simulink model "GNSS_MPCcontrolledSpacecraft"  (R2025b)
settings: Solver=ode113  StartTime=0.0  StopTime=120  FixedStep=1*60*60  RelTol=1e-8  AbsTol=1e-8
values from neighbouring files (symbols this model uses):
  area = 15    [Script_Concurso_Spacecraft_batch.m]    (also in initialize_inoas_simulation.m = 0.03)
  initMass = m_sat    (= 10000)    [Script_Concurso_Spacecraft_batch.m]    (also in initialize_inoas_simulation.m = 3.99)
  lamda_init = 1    [initialize_inoas_simulation.m]
  m = cfg.m    [MPC_INOAS.m]    (also in Script_Concurso_Spacecraft_batch.m = 3; initialize_inoas_simulation.m = 3)
  ref = 1.3    [Script_Concurso_Spacecraft_batch.m]    (also in initialize_inoas_simulation.m = 1)
  s = [sigma_x,sigma_x,sigma_x,sigma_v,sigma_v,sigma_v]    [Script_Concurso_Spacecraft_batch.m]    (also in initialize_inoas_simulation.m = [sigma_x, sigma_x, sigma_x, sigma_v, sigma_v, sigma_v])
  S_inv = inv(S)    [Script_Concurso_Spacecraft_batch.m]    (also in initialize_inoas_simulation.m)
  S_T_inv = inv(S')    [Script_Concurso_Spacecraft_batch.m]    (also in initialize_inoas_simulation.m)
  Ts = 1    [Script_Concurso_Spacecraft_batch.m]    (also in initialize_inoas_simulation.m)
  var_alt = sigma_alt^2    (= 1)    [Script_Concurso_Spacecraft_batch.m]    (also in initialize_inoas_simulation.m = 4000000)
  var_IMU = 0.01    [Script_Concurso_Spacecraft_batch.m]
  var_pos = sigma_pos^2    (= 10000)    [Script_Concurso_Spacecraft_batch.m]    (also in initialize_inoas_simulation.m = 4000000)
undefined symbols (not defined in the file or in its folder): endDate, thrustingThreshold
libraries: simulink x6, vrlib x2, sharedTrackingLibrary x1, aerolibsatdyn x1, aerolibutil x1
settings Model: SimulationMode=accelerator  Creator=benit  LastModifiedBy=Enrique Valverde

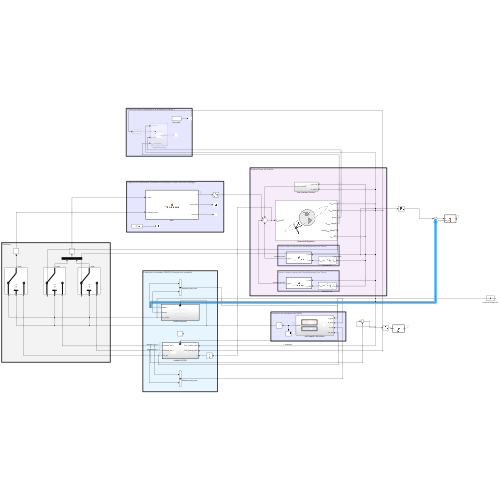
[thumbnail: Simulink's stored preview of the top-level diagram]
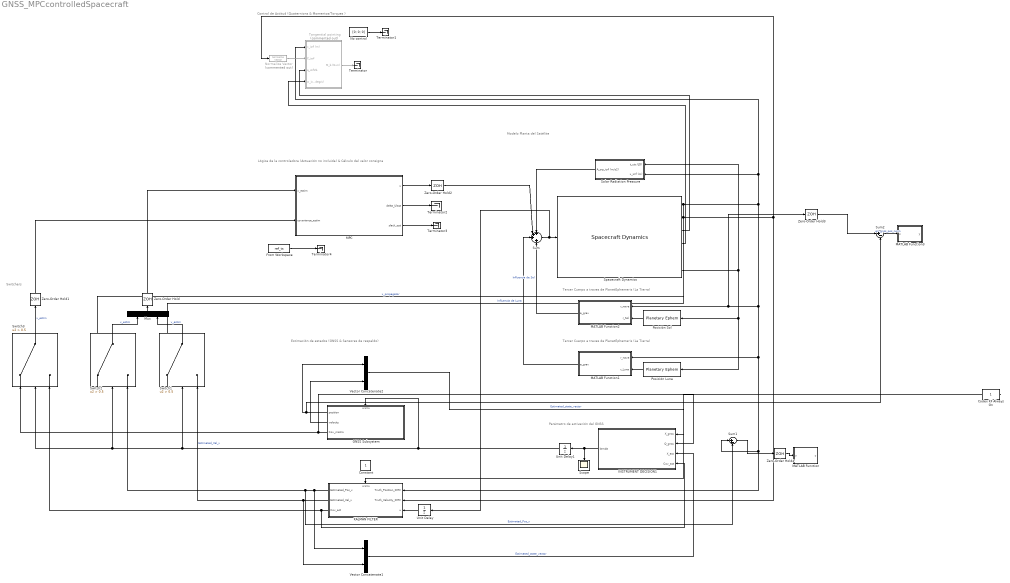
== system GNSS_MPCcontrolledSpacecraft ==
  note: Switchers
  note: Control de Actitud (Quaternions & Momentos/Torques )
  note: Lógica de la controladora (Actuación no incluida) & Cálculo del valor consigna
  note: Estimación de estados (GNSS & Sensores de respaldo)
  note: Parámetro de activación del GNSS
  note: Modelo Planta del Satélite
  note: Tercer Cuerpo a traves de PlanetEphemeris (La Tierra)
  note: Tercer Cuerpo a traves de PlanetEphemeris (La Tierra)
  Codex KF Always On : Constant  OutDataTypeStr=boolean
  Constant : Constant
  From Workspace : FromWorkspace  VariableName=ref_ts  SampleTime=1
  GNSS Subsystem : Subsystem  Description=|  TreatAsAtomicUnit=on
      | "GNSS ON"
      | 
      | Aquí va a ir las medidas del vector de estados utilizando GNSS. 
      | 
      | Se tendrá que añadir todo el sistema de ruido blanco del sensor, así como la regresión
      | por medio de mínimos cuadrados (WLSQ)
  INSTRUMENT DECISION1 : Subsystem
  KALMAN FILTER : Subsystem  Description=|  TreatAsAtomicUnit=on
      | "GNSS OFF"
      | 
      | Aquí va a ir las medidas del vector de estados utilizando Backup Sensor. 
      | 
      | Se tendrá que añadir todo el sistema de ruido blanco de los sensor de respaldo, 
      | así como el Filtro de Kalman y la estadística que permita mezclar las distintas medidas 
      | de distinta procedencia.
  MATLAB Function : MATLAB Function  TreatAsAtomicUnit=on
  MATLAB Function1 : MATLAB Function  TreatAsAtomicUnit=on
  MATLAB Function2 : MATLAB Function  TreatAsAtomicUnit=on
  MATLAB Function3 : MATLAB Function  TreatAsAtomicUnit=on
  MPC : MATLAB Function  TreatAsAtomicUnit=on
  Mux : Mux  Inputs=2
  No control : Constant  Value=[0; 0; 0]
  Normalize Vector : vrlib/Utilities/Normalize Vector  Commented=on  maxzero=0
  Posición Luna : PlanetaryEphem  units=m,m/s  center=Sun  startDate=startDate2  endDate=endDate*1.02  outputVelocity=off
  Posición Sol : PlanetaryEphem  units=m,m/s  target=Sun  startDate=startDate2  endDate=endDate*1.02  outputVelocity=off
  Scope : Scope
      settings: ActiveDisplayYMinimum=0.9  ActiveDisplayYMaximum=1.1
  Solar Radiation Pressure : Subsystem
  Spacecraft Dynamics : SpacecraftDynamics  forcesIn=off  momentsIn=off  accelIn=on  startDate=start_date  mass=m_sat  semiMajorAxis=a  eccentricity=ecc  inclination=inc  raan=RAAN  argPeriapsis=w  trueAnomaly=theta  outputAngAccel=on  shDegree=2  ephemerisStartDate=start_date  ephemerisEndDate=start_date
  Sum : Sum  Inputs=+++|+
  Sum1 : Sum  Inputs=|+-
  Sum2 : Sum  Inputs=|+-
  Switch1 : Switch  Criteria=u2 > Threshold  Threshold=0.5  SaturateOnIntegerOverflow=off  InputSameDT=off
  Switch2 : Switch  Criteria=u2 > Threshold  Threshold=0.5  SaturateOnIntegerOverflow=off  InputSameDT=off
  Switch3 : Switch  Criteria=u2 > Threshold  Threshold=0.5  SaturateOnIntegerOverflow=off  InputSameDT=off
  Tangential pointing : Subsystem  Commented=on
  Terminator{,1..4} (5 alike) : Terminator
  Unit Delay : UnitDelay  InitialCondition=zeros(3,1)  SampleTime=Ts  HasFrameUpgradeWarning=on
  Unit Delay1 : UnitDelay  InitialCondition=lamda_init  SampleTime=Ts  HasFrameUpgradeWarning=on
  Vector Concatenate1 : Concatenate
  Vector Concatenate2 : Concatenate
  Zero-Order Hold : ZeroOrderHold  SampleTime=Ts
  Zero-Order Hold1 : ZeroOrderHold  SampleTime=Ts
  Zero-Order Hold2 : ZeroOrderHold  SampleTime=Ts
  Zero-Order Hold3 : ZeroOrderHold
  Zero-Order Hold4 : ZeroOrderHold
  wires:
  Spacecraft Dynamics/1 -> Sum1/1, KALMAN FILTER/1(Truth_Position_ICRF), MATLAB Function1/1(r_nave), Zero-Order Hold3/1, MATLAB Function2/1(r_nave), Tangential pointing/1(x_icrf (m)), Solar Radiation Pressure/2(x_icrf (m)), Switch2/1  "x_propagator"
  Spacecraft Dynamics/6 -> Solar Radiation Pressure/1(t_utc (JD)), Posición Luna/1, Posición Sol/1
  Posición Sol/1 -> MATLAB Function2/2(r_Sol)
  Posición Luna/1 -> MATLAB Function1/2(r_Luna)
  Spacecraft Dynamics/2 -> Normalize Vector/1, KALMAN FILTER/2(Truth_Velocity_ICRF), Switch1/1
  Spacecraft Dynamics/4 -> Tangential pointing/4(w_icrf2b (deg/s))
  Spacecraft Dynamics/3 -> Tangential pointing/3(q_icrf2b)
  Normalize Vector/1 -> Tangential pointing/2(C_icrf)
  Tangential pointing/1(M_b (N-m)) -> Terminator/1
  No control/1 -> Terminator1/1
  Solar Radiation Pressure/1(A_srp_icrf (m/s2)) -> Sum/1
  MATLAB Function2/1(a_grav) -> Sum/4  "Influencia de Sol"
  MATLAB Function1/1(a_grav) -> Sum/3  "Influencia de Luna"
  Sum/1 -> Spacecraft Dynamics/1, Unit Delay/1
  KALMAN FILTER/3(Cov_act) -> INSTRUMENT DECISION1/4(Cov_act), Switch3/3
  Unit Delay/1 -> KALMAN FILTER/3(u)
  Switch2/1 -> Mux/1  "x_estim"
  Switch1/1 -> Mux/2  "v_estim"
  Mux/1 -> Zero-Order Hold/1
  MPC/1(u) -> Zero-Order Hold2/1
  MPC/2(delta_Ulast) -> Terminator2/1
  MPC/3(slack_opt) -> Terminator3/1
  Zero-Order Hold/1 -> MPC/1(x_estim)
  Zero-Order Hold1/1 -> MPC/2(covariance_estim)
  Zero-Order Hold2/1 -> Sum/2
  From Workspace/1 -> Terminator4/1
  Unit Delay1/1 -> GNSS Subsystem/Enable, Switch3/2, Switch2/2, Switch1/2
  GNSS Subsystem/1(position) -> Sum2/2, Vector Concatenate2/1
  GNSS Subsystem/2(velocity) -> Vector Concatenate2/2
  KALMAN FILTER/1(Estimated_Pos_x) -> Vector Concatenate1/1, Sum1/2, Switch2/3  "Estimated_Pos_x"
  KALMAN FILTER/2(Estimated_Vel_v) -> Vector Concatenate1/2, Switch1/3  "Estimated_Vel_v"
  Switch3/1 -> Zero-Order Hold1/1  "x_estim"
  GNSS Subsystem/3(Cov_matrix) -> Switch3/1, INSTRUMENT DECISION1/2(Q_gnss)
  INSTRUMENT DECISION1/1(lamda) -> Scope/1, Unit Delay1/1
  Vector Concatenate1/1 -> INSTRUMENT DECISION1/3(X_est)  "Estimated_state_vector"
  Vector Concatenate2/1 -> INSTRUMENT DECISION1/1(X_gnss)  "Estimated_state_vector"
  Codex KF Always On/1 -> KALMAN FILTER/Enable
  Sum2/1 -> MATLAB Function3/1(u)  "err_gnss_pos_norm"
  Zero-Order Hold3/1 -> Sum2/1
  Zero-Order Hold4/1 -> MATLAB Function/1(u)
  Sum1/1 -> Zero-Order Hold4/1

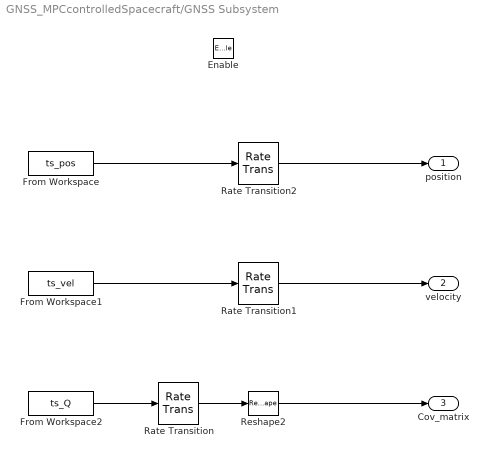
== system GNSS_MPCcontrolledSpacecraft/GNSS Subsystem ==
  Enable : EnablePort
  From Workspace : FromWorkspace  VariableName=ts_pos  SampleTime=Ts
  From Workspace1 : FromWorkspace  VariableName=ts_vel  SampleTime=Ts
  From Workspace2 : FromWorkspace  VariableName=ts_Q  SampleTime=Ts
  Rate Transition : RateTransition  InitialCondition=zeros(1,36)  OutPortSampleTime=Ts
  Rate Transition1 : RateTransition  InitialCondition=zeros(1,3)  OutPortSampleTime=Ts
  Rate Transition2 : RateTransition  InitialCondition=zeros(1,3)  OutPortSampleTime=Ts
  Reshape2 : Reshape  OutputDimensionality=Customize  OutputDimensions=[6 6]
  position : Outport  InitialOutput=zeros(3,1)
  velocity : Outport  Port=2  InitialOutput=zeros(3,1)
  Cov_matrix : Outport  Port=3  InitialOutput=zeros(6,6)
  wires:
  From Workspace1/1 -> Rate Transition1/1
  From Workspace2/1 -> Rate Transition/1
  Reshape2/1 -> Cov_matrix/1
  Rate Transition/1 -> Reshape2/1
  From Workspace/1 -> Rate Transition2/1
  Rate Transition2/1 -> position/1
  Rate Transition1/1 -> velocity/1

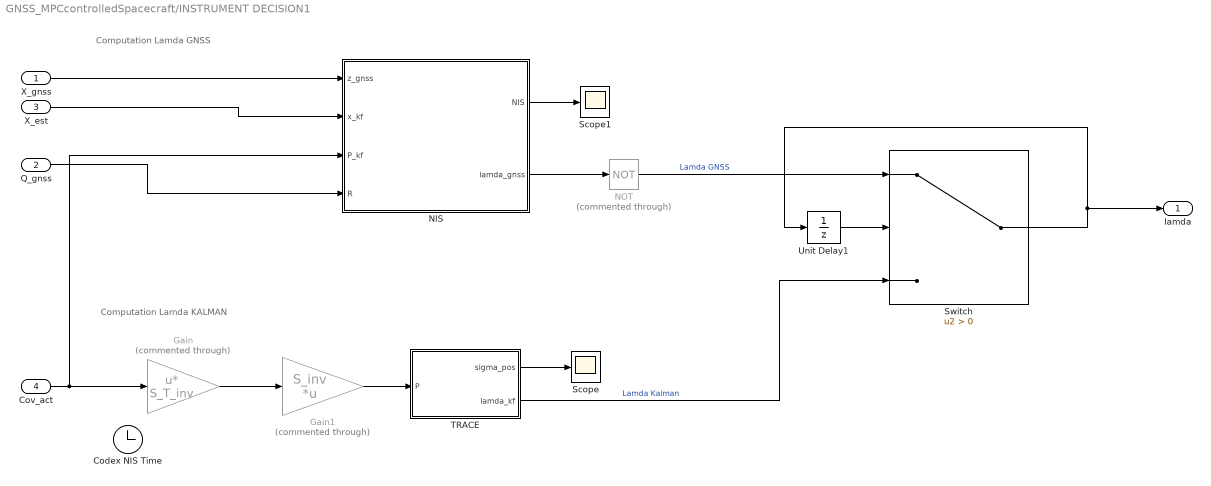
== system GNSS_MPCcontrolledSpacecraft/INSTRUMENT DECISION1 ==
  note: Computation Lamda GNSS
  note: Computation Lamda KALMAN
  X_gnss : Inport
  Q_gnss : Inport  Port=2
  X_est : Inport  Port=3
  Cov_act : Inport  Port=4
  Codex NIS Time : Clock
  Gain : Gain  Commented=through  Gain=S_T_inv  Multiplication=Matrix(u*K)
  Gain1 : Gain  Commented=through  Gain=S_inv  Multiplication=Matrix(K*u)
  NIS : MATLAB Function  TreatAsAtomicUnit=on
  NOT : Logic  Commented=through  Operator=NOT  IconShape=distinctive  AllPortsSameDT=off  OutDataTypeStr=boolean
  Scope : Scope
  Scope1 : Scope
      settings: DataLoggingVariableName=ScopeData2
  Switch : Switch  Criteria=u2 > Threshold  SaturateOnIntegerOverflow=off  InputSameDT=off
  TRACE : MATLAB Function  TreatAsAtomicUnit=on
  Unit Delay1 : UnitDelay  InitialCondition=lamda_init  SampleTime=Ts  HasFrameUpgradeWarning=on
  lamda : Outport
  wires:
  Gain/1 -> Gain1/1
  Gain1/1 -> TRACE/1(P)
  TRACE/1(sigma_pos) -> Scope/1
  NIS/2(lamda_gnss) -> NOT/1
  NIS/1(NIS) -> Scope1/1
  NOT/1 -> Switch/1  "Lamda GNSS"
  TRACE/2(lamda_kf) -> Switch/3  "Lamda Kalman"
  Switch/1 -> Unit Delay1/1, lamda/1
  Unit Delay1/1 -> Switch/2
  X_gnss/1 -> NIS/1(z_gnss)
  Q_gnss/1 -> NIS/4(R)
  X_est/1 -> NIS/2(x_kf)
  Cov_act/1 -> NIS/3(P_kf), Gain/1

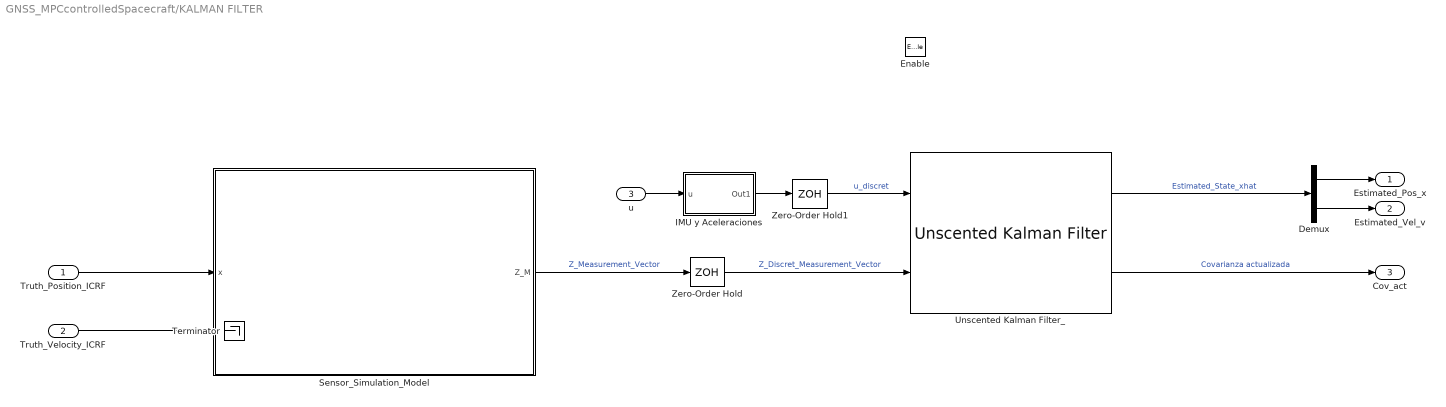
== system GNSS_MPCcontrolledSpacecraft/KALMAN FILTER ==
  Truth_Position_ICRF : Inport
  Truth_Velocity_ICRF : Inport  Port=2
  u : Inport  Port=3  PortDimensions=[3 1]
  Enable : EnablePort
  Demux : Demux  Outputs=2
  IMU y Aceleraciones : Subsystem
  Sensor_Simulation_Model : Subsystem
  Terminator : Terminator
  Unscented Kalman Filter_ : sharedTrackingLibrary/Unscented Kalman Filter  StateTransitionFcn=myStateTransitionFcn  HasAdditiveProcessNoise=Additive  ProcessNoise=Q_matrix  HasTimeVaryingProcessNoise=off  HasStateTransitionFcnExtraArgument=1  InitialState=x0_kalman  InitialStateCovariance=P0_kalman  Alpha=1e-3  Beta=2  Kappa=0  MeasurementFcn1=myMeasurementFcn  HasMeasurementEnablePort1=off  HasAdditiveMeasurementNoise1=Additive  MeasurementNoise1=R_matrix  HasTimeVaryingMeasurementNoise1=off  HasMeasurementFcnExtraArgument1=0  HasMeasurementWrapping1=off  MeasurementFcn2=myMeasurementFcn  HasMeasurementEnablePort2=off  HasAdditiveMeasurementNoise2=Additive  MeasurementNoise2=1  HasTimeVaryingMeasurementNoise2=off  HasMeasurementFcnExtraArgument2=0  HasMeasurementWrapping2=off  MeasurementFcn3=myMeasurementFcn  HasMeasurementEnablePort3=off  HasAdditiveMeasurementNoise3=Additive  MeasurementNoise3=1  HasTimeVaryingMeasurementNoise3=off  HasMeasurementFcnExtraArgument3=0  HasMeasurementWrapping3=off  MeasurementFcn4=myMeasurementFcn  HasMeasurementEnablePort4=off  HasAdditiveMeasurementNoise4=Additive  MeasurementNoise4=1  HasTimeVaryingMeasurementNoise4=off  HasMeasurementFcnExtraArgument4=0  HasMeasurementWrapping4=off  MeasurementFcn5=myMeasurementFcn  HasMeasurementEnablePort5=off  HasAdditiveMeasurementNoise5=Additive  MeasurementNoise5=1  HasTimeVaryingMeasurementNoise5=off  HasMeasurementFcnExtraArgument5=0  HasMeasurementWrapping5=off  EnableMultirate=off  StateTransitionFcnSampleTime=1  MeasurementFcn1SampleTime=1  MeasurementFcn2SampleTime=1  MeasurementFcn3SampleTime=1  MeasurementFcn4SampleTime=1  MeasurementFcn5SampleTime=1  UseCurrentEstimator=on  OutputStateCovariance=on  DataType=double  SampleTime=Ts  NumberOfMeasurements=1
      settings: LibrarySourceBlock=cstblocks/State Estimation/Unscented Kalman Filter
  Zero-Order Hold : ZeroOrderHold  SampleTime=Ts
  Zero-Order Hold1 : ZeroOrderHold  SampleTime=Ts
  Estimated_Pos_x : Outport  InitialOutput=zeros(3,1)
  Estimated_Vel_v : Outport  Port=2  InitialOutput=zeros(3,1)
  Cov_act : Outport  Port=3  InitialOutput=zeros(6,6)
  wires:
  Truth_Velocity_ICRF/1 -> Terminator/1
  Unscented Kalman Filter_/1 -> Demux/1  "Estimated_State_xhat"
  Unscented Kalman Filter_/2 -> Cov_act/1  "Covarianza actualizada"
  Truth_Position_ICRF/1 -> Sensor_Simulation_Model/1(x)
  Demux/1 -> Estimated_Pos_x/1
  Demux/2 -> Estimated_Vel_v/1
  Sensor_Simulation_Model/1(Z_M) -> Zero-Order Hold/1  "Z_Measurement_Vector"
  Zero-Order Hold/1 -> Unscented Kalman Filter_/2  "Z_Discret_Measurement_Vector"
  Zero-Order Hold1/1 -> Unscented Kalman Filter_/1  "u_discret"
  u/1 -> IMU y Aceleraciones/1(u)
  IMU y Aceleraciones/1(Out1) -> Zero-Order Hold1/1

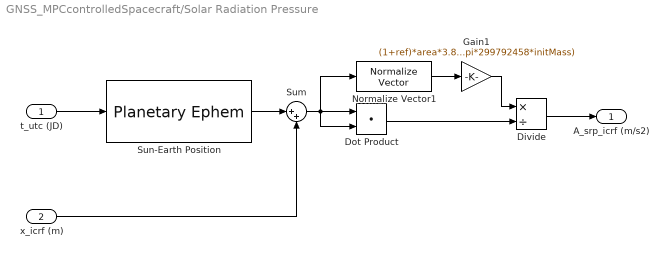
== system GNSS_MPCcontrolledSpacecraft/Solar Radiation Pressure ==
  t_utc (JD) : Inport
  x_icrf (m) : Inport  Port=2
  Divide : Product  Inputs=*/
  Dot Product : DotProduct  OutDataTypeStr=Inherit: Inherit via internal rule
  Gain1 : Gain  Gain=(1+ref)*area*3.852e26/(4*pi*299792458*initMass)
  Normalize Vector1 : vrlib/Utilities/Normalize Vector  maxzero=0
  Sum : Sum  Inputs=|++
  Sun-Earth Position : PlanetaryEphem  units=m,m/s  center=Sun  target=Earth  outputVelocity=off
  A_srp_icrf (m/s2) : Outport
  wires:
  Normalize Vector1/1 -> Gain1/1
  Gain1/1 -> Divide/1
  Dot Product/1 -> Divide/2
  Divide/1 -> A_srp_icrf (m/s2)/1
  t_utc (JD)/1 -> Sun-Earth Position/1
  Sun-Earth Position/1 -> Sum/1
  Sum/1 -> Dot Product/1, Normalize Vector1/1, Dot Product/2
  x_icrf (m)/1 -> Sum/2

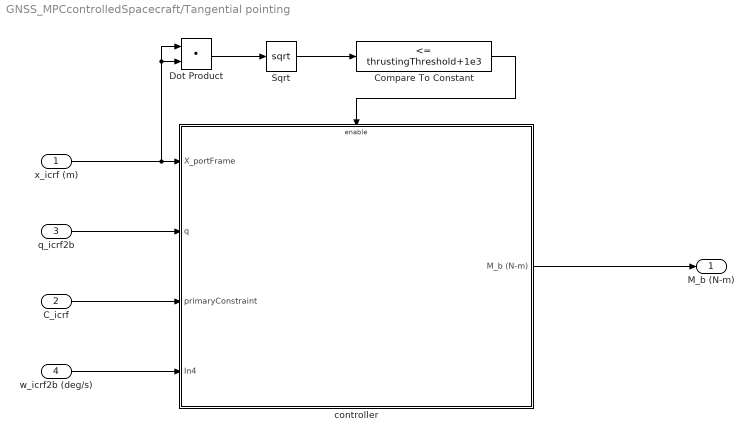
== system GNSS_MPCcontrolledSpacecraft/Tangential pointing ==
  x_icrf (m) : Inport
  C_icrf : Inport  Port=2
  q_icrf2b : Inport  Port=3
  w_icrf2b (deg/s) : Inport  Port=4
  Compare To Constant : simulink/Logic and Bit Operations/Compare To Constant  relop=<=  const=thrustingThreshold+1e3  OutDataTypeStr=boolean
  Dot Product : DotProduct  OutDataTypeStr=Inherit: Inherit via internal rule
  Sqrt : Sqrt
  controller : Subsystem
  M_b (N-m) : Outport
  wires:
  q_icrf2b/1 -> controller/2(q)
  C_icrf/1 -> controller/3(primaryConstraint)
  w_icrf2b (deg/s)/1 -> controller/4(In4)
  controller/1(M_b (N-m)) -> M_b (N-m)/1
  Dot Product/1 -> Sqrt/1
  Sqrt/1 -> Compare To Constant/1
  x_icrf (m)/1 -> Dot Product/1, Dot Product/2, controller/1(X_portFrame)
  Compare To Constant/1 -> controller/Enable

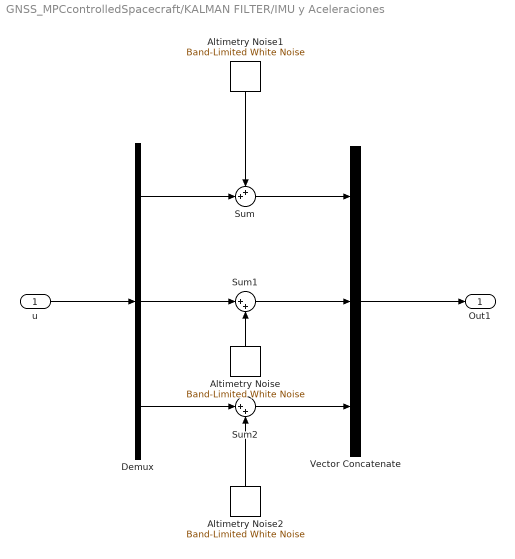
== system GNSS_MPCcontrolledSpacecraft/KALMAN FILTER/IMU y Aceleraciones ==
  u : Inport  PortDimensions=[3 1]
  Altimetry Noise : simulink/Sources/Band-Limited White Noise  Cov=var_IMU* Ts  Ts=Ts  seed=[23341]
  Altimetry Noise1 : simulink/Sources/Band-Limited White Noise  Cov=var_IMU* Ts  Ts=Ts  seed=[23341]
  Altimetry Noise2 : simulink/Sources/Band-Limited White Noise  Cov=var_IMU* Ts  Ts=Ts  seed=[23341]
  Demux : Demux  Outputs=3
  Sum : Sum  Inputs=++|
  Sum1 : Sum  Inputs=|++
  Sum2 : Sum  Inputs=|++
  Vector Concatenate : Concatenate  NumInputs=3
  Out1 : Outport
  wires:
  Vector Concatenate/1 -> Out1/1
  u/1 -> Demux/1
  Demux/1 -> Sum/2
  Altimetry Noise1/1 -> Sum/1
  Demux/3 -> Sum2/1
  Altimetry Noise2/1 -> Sum2/2
  Demux/2 -> Sum1/1
  Altimetry Noise/1 -> Sum1/2
  Sum/1 -> Vector Concatenate/1
  Sum2/1 -> Vector Concatenate/3
  Sum1/1 -> Vector Concatenate/2

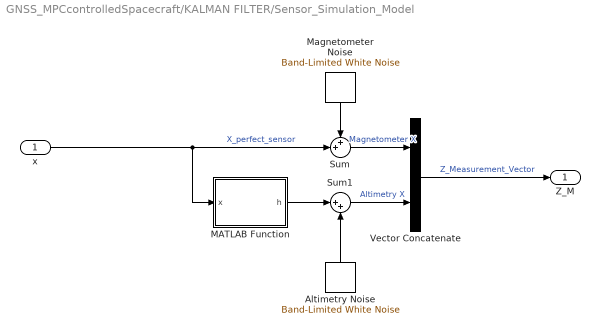
== system GNSS_MPCcontrolledSpacecraft/KALMAN FILTER/Sensor_Simulation_Model ==
  x : Inport
  Altimetry Noise : simulink/Sources/Band-Limited White Noise  Cov=var_alt* Ts  Ts=Ts  seed=[23341]
  MATLAB Function : MATLAB Function  TreatAsAtomicUnit=on
  Magnetometer Noise : simulink/Sources/Band-Limited White Noise  Cov=var_pos * Ts  Ts=Ts  seed=[23341]
  Sum : Sum  Inputs=++|
  Sum1 : Sum  Inputs=|++
  Vector Concatenate : Concatenate
  Z_M : Outport
  wires:
  x/1 -> MATLAB Function/1(x), Sum/2  "X_perfect_sensor"
  Altimetry Noise/1 -> Sum1/2
  Sum/1 -> Vector Concatenate/1  "Magnetometer X"
  MATLAB Function/1(h) -> Sum1/1
  Magnetometer Noise/1 -> Sum/1
  Sum1/1 -> Vector Concatenate/2  "Altimetry X"
  Vector Concatenate/1 -> Z_M/1  "Z_Measurement_Vector"

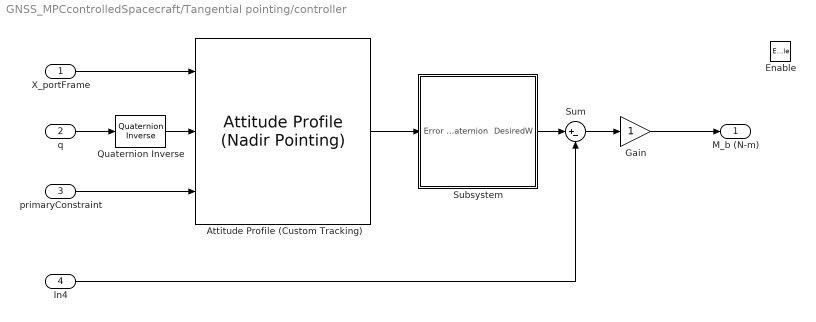
== system GNSS_MPCcontrolledSpacecraft/Tangential pointing/controller ==
  X_portFrame : Inport
  q : Inport  Port=2
  primaryConstraint : Inport  Port=3
  In4 : Inport  Port=4
  Enable : EnablePort
  Attitude Profile (Custom Tracking) : aerolibsatdyn/Attitude Profile (Nadir Pointing)  outputError=on  outputFinalAttitude=off  portFrame=ICRF  pointingMode=Custom  celestialTarget=Sun  tunablePointing=off  primaryAlignmentSrc=Dialog  primaryAlignment=[1 0 0]  secondaryAlignmentSrc=Dialog  secondaryAlignment=[0 0 1]  constraintFrame=ICRF  primaryConstraintSrc=Port  primaryConstraint=[1 0 0]  secondaryConstraintSrc=Dialog  secondaryConstraint=[0 0 1]
      settings: LibrarySourceBlock=|
      | aerolibsatdyn/Attitude Profile
      | (Sun Tracking)
  Gain : Gain
  Quaternion Inverse : aerolibutil/Quaternion Inverse
  Subsystem : Subsystem
  Sum : Sum  Inputs=|+-
  M_b (N-m) : Outport
  wires:
  X_portFrame/1 -> Attitude Profile (Custom Tracking)/1
  Sum/1 -> Gain/1
  primaryConstraint/1 -> Attitude Profile (Custom Tracking)/3
  Quaternion Inverse/1 -> Attitude Profile (Custom Tracking)/2
  Attitude Profile (Custom Tracking)/1 -> Subsystem/1(Error quaternion)
  Gain/1 -> M_b (N-m)/1
  Subsystem/1(DesiredW) -> Sum/1
  In4/1 -> Sum/2
  q/1 -> Quaternion Inverse/1

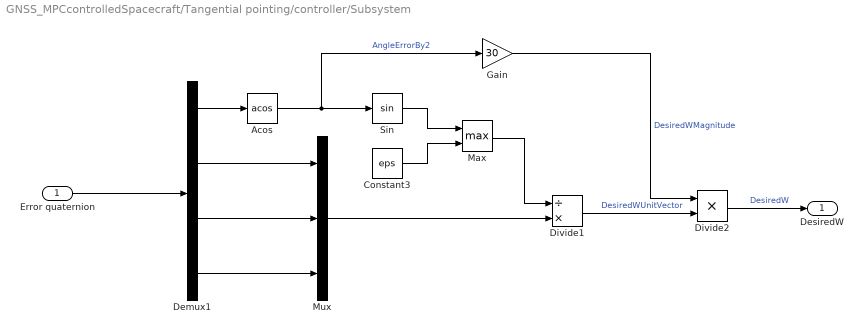
== system GNSS_MPCcontrolledSpacecraft/Tangential pointing/controller/Subsystem ==
  Error quaternion : Inport
  Acos : Trigonometry  Operator=acos
  Constant3 : Constant  Value=eps
  Demux1 : Demux
  Divide1 : Product  Inputs=/*
  Divide2 : Product  Inputs=**
  Gain : Gain  Gain=30
  Max : MinMax  Function=max  Inputs=2
  Mux : Mux  Inputs=3
  Sin : Trigonometry
  DesiredW : Outport
  wires:
  Error quaternion/1 -> Demux1/1
  Gain/1 -> Divide2/1  "DesiredWMagnitude"
  Demux1/2 -> Mux/1
  Demux1/1 -> Acos/1
  Acos/1 -> Sin/1, Gain/1  "AngleErrorBy2"
  Mux/1 -> Divide1/2
  Divide2/1 -> DesiredW/1  "DesiredW"
  Constant3/1 -> Max/2
  Demux1/3 -> Mux/2
  Max/1 -> Divide1/1
  Demux1/4 -> Mux/3
  Sin/1 -> Max/1
  Divide1/1 -> Divide2/2  "DesiredWUnitVector"

== matlab function GNSS_MPCcontrolledSpacecraft/MATLAB Function1 ==
  data: r_nave input; a_grav output; r_Luna input
function a_grav = gravedadLuna(r_nave, r_Luna)
%#codegen

% Constante gravitacional de Marte
mu_Luna = 4.90e12; % [m^3/s^2]

% Vector relativo
r_rel = r_nave - r_Luna;

% Magnitud de la distancia
dist = norm(r_rel);

% Aceleración gravitatoria
a_grav = (-mu_Luna / dist^3) * r_rel;

end

== matlab function GNSS_MPCcontrolledSpacecraft/KALMAN FILTER/Sensor_Simulation_Model/MATLAB Function ==
  data: x input; h output
function h = altimetry(x)
% Cálculo de la distancia radial
R_Tierra= 6378137.0;       % Radio ecuatorial [m]
h=sqrt((x(1)^2)+(x(2)^2)+(x(3)^2))-R_Tierra;

== matlab function GNSS_MPCcontrolledSpacecraft/MATLAB Function2 ==
  data: r_nave input; a_grav output; r_Sol input
function a_grav = gravedadSol(r_nave, r_Sol)
%#codegen

% Constante gravitacional de Marte
mu_sol = 1.327e20; % [m^3/s^2]

% Vector relativo
r_rel = r_nave - r_Sol;

% Magnitud de la distancia
dist = norm(r_rel);

% Aceleración gravitatoria
a_grav = (-mu_sol / dist^3) * r_rel;

end

== matlab function GNSS_MPCcontrolledSpacecraft/MATLAB Function ==
  data: u input; y output
function y = fcn(u)
y = norm(u);

== matlab function GNSS_MPCcontrolledSpacecraft/MPC ==
  data: x_estim input; u output; covariance_estim input; delta_Ulast output; slack_opt output
function [u, delta_Ulast, slack_opt] = MPC_INOAS_block(x_estim, covariance_estim)

%#codegen
coder.extrinsic('MPC_INOAS');

u = zeros(3,1);
delta_Ulast = zeros(120,1);
slack_opt = zeros(40,1);

[u_tmp, delta_tmp, slack_tmp] = MPC_INOAS(x_estim, covariance_estim);

u = u_tmp;
delta_Ulast = delta_tmp;
slack_opt = slack_tmp;

end

== matlab function GNSS_MPCcontrolledSpacecraft/INSTRUMENT DECISION1/NIS ==
  data: NIS output; z_gnss input; lamda_gnss output; x_kf input; P_kf input; R input
function [NIS, lamda_gnss] = compute_NIS(z_gnss, x_kf, P_kf, R)
persistent good_count
if isempty(good_count)
    good_count = 0;
end

nu = z_gnss - x_kf;
S  = 0.5*(P_kf + P_kf.') + 0.5*(R + R.');
S  = S + 1e-9*eye(6);

NIS = nu' * (S \ nu);

% Umbral inicial de trabajo.
% Si luego hacéis coherente z_gnss con R, podéis volver a 12.59.
nis_enter = 25;
N_good    = 10;

if NIS < nis_enter
    good_count = good_count + 1;
else
    good_count = 0;
end

if good_count >= N_good
    lamda_gnss = 0;   % pasar a KF
else
    lamda_gnss = 1;   % seguir en GNSS
end
end

== matlab function GNSS_MPCcontrolledSpacecraft/INSTRUMENT DECISION1/TRACE ==
  data: sigma_pos output; P input; lamda_kf output
function [sigma_pos, lamda_kf] = fcn(P)
Pr = P(1:3,1:3);
Pr = 0.5*(Pr + Pr.');

sigma_pos = sqrt(max(trace(Pr), 0));

% Tuning inicial
sigma_high = 50;   % [m]

if sigma_pos >= sigma_high
    lamda_kf = 1;   % volver a GNSS
else
    lamda_kf = 0;   % quedarse en KF
end
end

== matlab function GNSS_MPCcontrolledSpacecraft/MATLAB Function3 ==
  data: u input; y output
function y = fcn(u)
y = norm(u);
